simulink model "PubIfDecisionLSM_MDL"  (R2020b)
settings: configuration reference "DspaceConfig" (kept outside this file)
PostLoadFcn:
  | if any(exist('dsrtsu_mdlpostloadfcn', 'file') ~= 0), dsrtsu_mdlpostloadfcn('Execute', bdroot); end
InitFcn:
  | , if any(exist('rtifpga_mdlclblib', 'file') ~= 0), rtifpga_mdlclblib('Init', bdroot); end,
  | , if any(exist('dsmpb_private', 'file') ~= 0), dsmpb_private('dsmpb_mdlclblib', 'Init', bdroot); end,
values from neighbouring files (symbols this model uses):
  P_LSM_ALC_Enable = 0.0    [LSM_Parameter.sldd]
  P_LSM_AwayEdge_offset = 0.1    [LSM_Parameter.sldd]
  P_LSM_CentValidErr = 1.0    [LSM_Parameter.sldd]
  P_LSM_DOP_C0_EN_Limit = 0.8    [LSM_Parameter.sldd]
  P_LSM_DOP_C0_out_Limit = 2.0    [LSM_Parameter.sldd]
  P_LSM_DOP_C1_EN_Limit : value not decoded    [LSM_Parameter.sldd]
  P_LSM_DOP_C1_out_Limit : value not decoded    [LSM_Parameter.sldd]
  P_LSM_DOP_C1AndC2_Lim_X : value not decoded    [LSM_Parameter.sldd]
  P_LSM_DOP_C2_EN_Limit : value not decoded    [LSM_Parameter.sldd]
  P_LSM_DOP_C2_out_Limit : value not decoded    [LSM_Parameter.sldd]
  P_LSM_DOP_In_Pre2Dop_Dis = 1.0    [LSM_Parameter.sldd]
  P_LSM_DOP_Out_Pre2Dop_Dis = 2.0    [LSM_Parameter.sldd]
  P_LSM_DOP_PreDis_X : value not decoded    [LSM_Parameter.sldd]
  P_LSM_DOP_PreDis_Y : value not decoded    [LSM_Parameter.sldd]
  P_LSM_DOPEnableSW = 1.0    [LSM_Parameter.sldd]
  P_LSM_DOPValid_CheckTime = 0.06    [LSM_Parameter.sldd]
  P_LSM_DoubleLine_Curr2Cent_Dislimit = 0.5    [LSM_Parameter.sldd]
  P_LSM_DoubleLine_Dop2Cent_Dislimit = 0.5    [LSM_Parameter.sldd]
  P_LSM_DoubleLine_DOPOut_C1 : value not decoded    [LSM_Parameter.sldd]
  P_LSM_DoubleLine_Pre2Cent_Dislimit = 1.0    [LSM_Parameter.sldd]
  P_LSM_Error_Limit = 0.5    [LSM_Parameter.sldd]
  P_LSM_IFV2CenterAxis = 0.0    [LSM_Parameter.sldd]
  P_LSM_IFV2RearAxis = 0.0    [LSM_Parameter.sldd]
  P_LSM_Line2Edge_limit = 0.5    [LSM_Parameter.sldd]
  P_LSM_Line_Error = 0.1    [LSM_Parameter.sldd]
  P_LSM_LineSTD_Limit = 0.15    [LSM_Parameter.sldd]
  P_LSM_NOH_Switch = 0.0    [LSM_Parameter.sldd]
  P_LSM_OTL_C0_Factor = 1.0    [LSM_Parameter.sldd]
  P_LSM_OTL_C1_Factor = 0.5    [LSM_Parameter.sldd]
  P_LSM_OTL_C2_Factor = 0.5    [LSM_Parameter.sldd]
  P_LSM_Pre2OnlyLineDis = 5.0    [LSM_Parameter.sldd]
  P_LSM_Pre_t = 0.0    [LSM_Parameter.sldd]
  P_LSM_SingleLine_Cent2Edge_Dislimit = 100.0    [LSM_Parameter.sldd]
  P_LSM_SingleLine_Curr2Cent_Dislimit = 0.2    [LSM_Parameter.sldd]
  P_LSM_SingleLine_Dop2Cent_Dislimit = 0.2    [LSM_Parameter.sldd]
  P_LSM_SingleLine_DOPOut_C1 : value not decoded    [LSM_Parameter.sldd]
  P_LSM_SingleLine_Pre2Cent_Dislimit = 0.5    [LSM_Parameter.sldd]
  P_LSM_TJALimitSpd = 60.0    [LSM_Parameter.sldd]
undefined symbols (not defined in the file or in its folder): P_lCS_IFV2CenterAxis, P_LCS_IFV2RearAxis, P_LSM_EntryEdge_offset, P_LSM_EntryLnChngEnSwitch, P_LSM_EntryVanishDis, P_LSM_LinetLostTime, P_LSM_LineWijCal_C12, P_LSM_LineWijCal_C13, P_LSM_MapValid_ErrorSwitch, P_LSM_PosLineLcFac, P_LSM_SpdLim_Stub_Spd, P_LSM_SpdLim_StubLength, P_LSM_SpdTurnAlarm
libraries: simulink x324, TrueDurationTime x11
(part 15 of 25)

== matlab function PubIfDecisionLSM_MDL/Subsystem1/TargetLineCalc_20ms/TargetLineCalc/MATLAB Function4 ==
  data: LH1Wij input; LH2Wij input; LH1_Valid input; LH2_Valid input; CentLineValid output; VisLineConf input; VisLineA3 input; VisLineA2 input; VisLineA1 input; VisLineA0 input; VisLineR input; RoadWidth input; CentLineC3 output; CentLineC2 output; CentLineC1 output; CentLineC0 output; CentLineRange output; CentLineReliable output; LeftLineValid output; LeftLineC3 output; LeftLineC2 output; LeftLineC1 output; LeftLineC0 output; LeftLineRange output; LeftLineReliable output; LeftLaneAvail output; RightLineValid output; RightLineC3 output; RightLineC2 output; RightLineC1 output; RightLineC0 output; RightLineRange output; RightLineReliable output; RightLaneAvail output; Line_State output; preDis input
function [CentLineValid,CentLineC3,CentLineC2,CentLineC1,CentLineC0,CentLineRange,CentLineReliable,...
    LeftLineValid,LeftLineC3,LeftLineC2,LeftLineC1,LeftLineC0,LeftLineRange,LeftLineReliable,LeftLaneAvail,...
    RightLineValid,RightLineC3,RightLineC2,RightLineC1,RightLineC0,RightLineRange,RightLineReliable,RightLaneAvail,...
    Line_State] = ...
    VisFilter(LH1Wij,LH2Wij,LH1_Valid,LH2_Valid,...
    VisLineConf,VisLineA3,VisLineA2,VisLineA1,VisLineA0,VisLineR,RoadWidth,preDis)

CentLineValid = false;
CentLineC0 = single(0);
CentLineC1 = single(0);
CentLineC2 = single(0);
CentLineC3 = single(0);
CentLineRange = single(0);
CentLineReliable = single(0);
Line_State = uint8(0);

if (LH1_Valid) && (LH2_Valid)
    Range_Error = VisLineR(2) - VisLineR(3);
    LH1_Offset = single(0.5);
    LH2_Offset = single(0.5);
    if Range_Error>10 || Range_Error<-10
        LH1_Offset = 0.5+min(0.5,Range_Error*0.01);
        LH2_Offset = 1-LH1_Offset;
    end
    CentLineValid = true;
    CentLineC0 = 0.5*(VisLineA0(2) + VisLineA0(3));
    CentLineC1 = LH1_Offset*VisLineA1(2) + LH2_Offset*VisLineA1(3);
    CentLineC2 = LH1_Offset*VisLineA2(2) + LH2_Offset*VisLineA2(3);
    CentLineC3 = LH1_Offset*VisLineA3(2) + LH2_Offset*VisLineA3(3);
    CentLineRange = max(VisLineR(2),VisLineR(3));
    CentLineReliable = 0.5*(LH1Wij+LH2Wij);
    Line_State = uint8(3);
elseif LH1_Valid
    CentLineValid = true;
    CentLineC0 = VisLineA0(2)-0.5*RoadWidth*sqrt(1+VisLineA1(2)*VisLineA1(2));
    CentLineC1 = VisLineA1(2);
    CentLineC2 = VisLineA2(2);
    CentLineC3 = VisLineA3(2);
    CentLineRange = VisLineR(2);
    CentLineReliable = LH1Wij;
    Line_State = uint8(1);
elseif LH2_Valid
    CentLineValid = true;
    CentLineC0 = VisLineA0(3)+0.5*RoadWidth*sqrt(1+VisLineA1(3)*VisLineA1(3));
    CentLineC1 = VisLineA1(3);
    CentLineC2 = VisLineA2(3);
    CentLineC3 = VisLineA3(3);
    CentLineRange = VisLineR(3);
    CentLineReliable = LH2Wij;
    Line_State = uint8(2);
end

if LH1Wij>=0.3
    LeftLineValid = true;
    LeftLineC0 = VisLineA0(2) + 0.5*RoadWidth*sqrt(1+VisLineA1(2)*VisLineA1(2));
    LeftLineC1 = VisLineA1(2);
    LeftLineC2 = VisLineA2(2);
    LeftLineC3 = VisLineA3(2);
    LeftLineRange = VisLineR(2);
    LeftLineReliable = LH1Wij;
    t1 = VisLineA0(1)+VisLineA1(1)*preDis+VisLineA2(1)*preDis^2+VisLineA3(1)*preDis^3;
    t2 = VisLineA0(2)+VisLineA1(2)*preDis+VisLineA2(2)*preDis^2+VisLineA3(2)*preDis^3; 
    if (VisLineConf(1)>0)&&...
            ((VisLineA0(1)-VisLineA0(2))>3)&&...
            ((VisLineA0(1)-VisLineA0(2))<5.5)&&...
            ((t1 - t2)>3)
        LeftLaneAvail = true;
    else
        LeftLaneAvail = false;
    end
else
    LeftLineValid = false;
    LeftLineC0 = single(0);
    LeftLineC1 = single(0);
    LeftLineC2 = single(0);
    LeftLineC3 = single(0);
    LeftLineRange = single(0);
    LeftLineReliable = single(0);
    LeftLaneAvail = false;
end

if LH2Wij>=0.3
    RightLineValid = true;
    RightLineC0 = VisLineA0(3) - 0.5*RoadWidth*sqrt(1+VisLineA1(3)*VisLineA1(3));
    RightLineC1 = VisLineA1(3);
    RightLineC2 = VisLineA2(3);
    RightLineC3 = VisLineA3(3);
    RightLineRange = VisLineR(3);
    RightLineReliable = LH2Wij;
    
    t3 = VisLineA0(3)+VisLineA1(3)*preDis+VisLineA2(3)*preDis^2+VisLineA3(3)*preDis^3;
    t4 = VisLineA0(4)+VisLineA1(4)*preDis+VisLineA2(4)*preDis^2+VisLineA3(4)*preDis^3;

    if (VisLineConf(4)>0)&&...
            ((VisLineA0(3)-VisLineA0(4))>3)&&...
            ((VisLineA0(3)-VisLineA0(4))<5.5)&&...
            ((t3 - t4)>3)

        RightLaneAvail = true;
    else
        RightLaneAvail = false;
    end
else
    RightLineValid = false;
    RightLineC0 = single(0);
    RightLineC1 = single(0);
    RightLineC2 = single(0);
    RightLineC3 = single(0);
    RightLineRange = single(0);
    RightLineReliable = single(0);
    RightLaneAvail = false;
end

== matlab function PubIfDecisionLSM_MDL/Subsystem1/TargetLineCalc_20ms/TargetLineCalc/NOA ==
  data: LeftEn input boolean size=1; RightEn input boolean size=1; RFM_LineL1_Valid input uint8 size=1; RFM_LineL1_A0 input single size=1; RFM_LineL1_A1 input single size=1; RFM_LineL1_A2 input single size=1; RFM_LineL1_A3 input single size=1; RFM_LineL1_Range input single size=1; RFM_LineL2_Valid input uint8 size=1; RFM_LineL2_A0 input single size=1; RFM_LineL2_A1 input single size=1; RFM_LineL2_A2 input single size=1; RFM_LineL2_A3 input single size=1; RFM_LineL2_Range input single size=1; RFM_LineR1_Valid input uint8 size=1; RFM_LineR1_A0 input single size=1; RFM_LineR1_A1 input single size=1; RFM_LineR1_A2 input single size=1; RFM_LineR1_A3 input single size=1; RFM_LineR1_Range input single size=1; RFM_LineR2_Valid input uint8 size=1; RFM_LineR2_A0 input single size=1; RFM_LineR2_A1 input single size=1; RFM_LineR2_A2 input single size=1; RFM_LineR2_A3 input single size=1; RFM_LineR2_Range input single size=1; Exit_Valid input uint8 size=1; Exit_A0 input single size=1; Exit_A1 input single size=1; Exit_A2 input single size=1; Exit_A3 input single size=1; Exit_Range input single size=1; Exit_Start input; RFM_LineCL_Valid input uint8 size=1; RFM_LineCL_A0 input single size=1; RFM_LineCL_A1 input single size=1; RFM_LineCL_A2 input single size=1; RFM_LineCL_A3 input single size=1; RFM_LineCL_Range input single size=1; HWASts input uint8 size=1; HWAStsK1 input uint8 size=1; PilotSts input uint8 size=1; LaneChange input uint8 size=1; PilotRoadSts input uint8 size=1; DistanceLim input single size=1; HWALineValid output boolean size=1; MoveIDK1 input int8 size=1; HWALineC3 output single size=1; HWALineC2 output single size=1; HWALineC1 output single size=1; HWALineC0 output single size=1; HWARange output single size=1; HWALeLineValid output boolean size=1; HWALeLineC3 output single size=1; HWALeLineC2 output single size=1; HWALeLineC1 output single size=1; HWALeLineC0 output single size=1; HWALeRange output single size=1; HWARiLineValid output boolean size=1; HWARiLineC3 output single size=1; HWARiLineC2 output single size=1; HWARiLineC1 output single size=1; HWARiLineC0 output single size=1; HWARiRange output single size=1; MoveID output int8 size=1; LockIDK1 input int8 size=1; LockID output int8 size=1; Lock_counterK1 input uint8; Lock_counter output uint8
function [HWALineValid,HWALineC3,HWALineC2,HWALineC1,HWALineC0,HWARange,...
    HWALeLineValid,HWALeLineC3,HWALeLineC2,HWALeLineC1,HWALeLineC0,HWALeRange,...
    HWARiLineValid,HWARiLineC3,HWARiLineC2,HWARiLineC1,HWARiLineC0,HWARiRange,...
    MoveID,LockID,Lock_counter] = fcn(LeftEn,RightEn,RFM_LineL1_Valid,RFM_LineL1_A0,RFM_LineL1_A1,RFM_LineL1_A2,RFM_LineL1_A3,RFM_LineL1_Range,...
    RFM_LineL2_Valid,RFM_LineL2_A0,RFM_LineL2_A1,RFM_LineL2_A2,RFM_LineL2_A3,RFM_LineL2_Range,...
    RFM_LineR1_Valid,RFM_LineR1_A0,RFM_LineR1_A1,RFM_LineR1_A2,RFM_LineR1_A3,RFM_LineR1_Range,...
    RFM_LineR2_Valid,RFM_LineR2_A0,RFM_LineR2_A1,RFM_LineR2_A2,RFM_LineR2_A3,RFM_LineR2_Range,...
    Exit_Valid,Exit_A0,Exit_A1,Exit_A2,Exit_A3,Exit_Range,Exit_Start,...
    RFM_LineCL_Valid,RFM_LineCL_A0,RFM_LineCL_A1,RFM_LineCL_A2,RFM_LineCL_A3,RFM_LineCL_Range,HWASts,HWAStsK1,...
    PilotSts,LaneChange,PilotRoadSts,DistanceLim,MoveIDK1,LockIDK1,Lock_counterK1)
HWALineValid = false;
HWALineC3 = single(0);
HWALineC2 = single(0);
HWALineC1 = single(0);
HWALineC0 = single(0);
HWARange = single(0);

HWALeLineValid = false;
HWALeLineC3 = single(0);
HWALeLineC2 = single(0);
HWALeLineC1 = single(0);
HWALeLineC0 = single(0);
HWALeRange = single(0);

HWARiLineValid = false;
HWARiLineC3 = single(0);
HWARiLineC2 = single(0);
HWARiLineC1 = single(0);
HWARiLineC0 = single(0);
HWARiRange = single(0);

MoveID = MoveIDK1;
LockID = LockIDK1;
Lock_counter = max(Lock_counterK1-uint8(1),uint8(0));
if Lock_counter==0
    LockID = int8(0);
end

if (HWASts==1)||(HWASts==7)||(HWASts==0)||HWASts==2
    MoveID = int8(0);
end
Error=false;

%% NOH
if PilotSts~=0
    if HWASts==1||HWASts==2
        if RFM_LineCL_Valid>0
            HWALineValid = true;
            HWALineC3 = RFM_LineCL_A3;
            HWALineC2 = RFM_LineCL_A2;
            HWALineC1 = RFM_LineCL_A1;
            HWALineC0 = RFM_LineCL_A0;
            HWARange = RFM_LineCL_Range;
        end
        if RFM_LineL1_Valid>0&&RFM_LineL2_Valid>0&&...
                (RFM_LineL1_Range>DistanceLim||RFM_LineL2_Range>DistanceLim)&&LeftEn
            HWALeLineValid = true;
            HWALeLineC3 = 0.5*(RFM_LineL1_A3+RFM_LineL2_A3);
            HWALeLineC2 = 0.5*(RFM_LineL1_A2+RFM_LineL2_A2);
            HWALeLineC1 = 0.5*(RFM_LineL1_A1+RFM_LineL2_A1);
            HWALeLineC0 = 0.5*(RFM_LineL1_A0+RFM_LineL2_A0);
            HWALeRange = 0.5*(RFM_LineL1_Range+RFM_LineL2_Range);
        end
        if RFM_LineR1_Valid>0&&RFM_LineR2_Valid>0&&...
                (RFM_LineR1_Range>DistanceLim||RFM_LineR2_Range>DistanceLim)&&RightEn
            HWARiLineValid = true;
            HWARiLineC3 = 0.5*(RFM_LineR1_A3+RFM_LineR2_A3);
            HWARiLineC2 = 0.5*(RFM_LineR1_A2+RFM_LineR2_A2);
            HWARiLineC1 = 0.5*(RFM_LineR1_A1+RFM_LineR2_A1);
            HWARiLineC0 = 0.5*(RFM_LineR1_A0+RFM_LineR2_A0);
            HWARiRange = 0.5*(RFM_LineR1_Range+RFM_LineR2_Range);
        end
    end
    if PilotRoadSts==8&&Exit_Valid           %汇出（未行驶到汇出线）
        if Exit_Start>30
            HWALineValid = true;
            HWALineC3 = RFM_LineCL_A3;
            HWALineC2 = RFM_LineCL_A2;
            HWALineC1 = RFM_LineCL_A1;
            HWALineC0 = RFM_LineCL_A0;
            HWARange = RFM_LineCL_Range;
        elseif Exit_Start>16
            temp_x = [0.5*Exit_Start,Exit_Start,Exit_Start+single(10),Exit_Start+single(30)];
            y1 = RFM_LineCL_A0+RFM_LineCL_A1*temp_x(1)+RFM_LineCL_A2*temp_x(1)^2+RFM_LineCL_A3*temp_x(1)^3;
            y3 = Exit_A0+Exit_A1*temp_x(3)+Exit_A2*temp_x(3)^2+Exit_A3*temp_x(3)^3;
            if y3>0
                y2 = min(1,0.4*y3);
            else
                y2 = max(-1,0.4*y3);
            end
            y4 = Exit_A0+Exit_A1*temp_x(4)+Exit_A2*temp_x(4)^2+Exit_A3*temp_x(4)^3;
            temp_y = [y1,y2,y3,y4];
            [HWALineC3,HWALineC2,HWALineC1,HWALineC0] = pl(temp_x,temp_y);
            HWALineValid = true;
            HWARange = Exit_Start+single(40);
        else
            HWALineValid = true;
            HWALineC3 = Exit_A3;
            HWALineC2 = Exit_A2;
            HWALineC1 = Exit_A1;
            HWALineC0 = Exit_A0;
            HWARange = Exit_Range;
        end
    elseif PilotRoadSts==19&&Exit_Valid         % 汇出（行驶到汇出线）
        HWALineValid = true;
        HWALineC3 = Exit_A3;
        HWALineC2 = Exit_A2;
        HWALineC1 = Exit_A1;
        HWALineC0 = Exit_A0;
        HWARange = Exit_Range;
    elseif HWASts==3 || HWASts==11 || HWASts==12       %巡航
        MoveID = int8(0);
        if HWAStsK1==5 || HWAStsK1==6
            Lock_counter = uint8(250);
            LockID = int8(0);
        end
        if Lock_counter>0
            if LaneChange==1
                LockID = LockID + int8(1);
            end
            if LaneChange==2
                LockID = LockID - int8(1);
            end
        else
            LockID = int8(0);
        end
        if LockID==1
            if RFM_LineR1_Valid>0&&RFM_LineR2_Valid>0&&...
                    (RFM_LineR1_Range>DistanceLim||RFM_LineR2_Range>DistanceLim)
                HWALineValid = true;
                HWALineC3 = 0.5*(RFM_LineR1_A3+RFM_LineR2_A3);
                HWALineC2 = 0.5*(RFM_LineR1_A2+RFM_LineR2_A2);
                HWALineC1 = 0.5*(RFM_LineR1_A1+RFM_LineR2_A1);
                HWALineC0 = 0.5*(RFM_LineR1_A0+RFM_LineR2_A0);
                HWARange = 0.5*(RFM_LineR1_Range+RFM_LineR2_Range);
            elseif RFM_LineR1_Valid>0&&...
                    RFM_LineR1_Range>DistanceLim
                HWALineValid = true;
                HWALineC3 = RFM_LineR1_A3;
                HWALineC2 = RFM_LineR1_A2;
                HWALineC1 = RFM_LineR1_A1;
                HWALineC0 = RFM_LineR1_A0 - 1.875*sqrt(single(1) + RFM_LineR1_A1*RFM_LineR1_A1);
                HWARange = RFM_LineR1_Range;
            elseif RFM_LineR2_Valid>0&&...
                    RFM_LineR2_Range>DistanceLim
                HWALineValid = true;
                HWALineC3 = RFM_LineR2_A3;
                HWALineC2 = RFM_LineR2_A2;
                HWALineC1 = RFM_LineR2_A1;
                HWALineC0 = RFM_LineR2_A0 + 1.875*sqrt(single(1) + RFM_LineR2_A1*RFM_LineR2_A1);
                HWARange = RFM_LineR2_Range;
            end
        elseif LockID==-1
            if RFM_LineL1_Valid>0&&RFM_LineL2_Valid>0&&...
                    (RFM_LineL1_Range>DistanceLim||RFM_LineL2_Range>DistanceLim)
                HWALineValid = true;
                HWALineC3 = 0.5*(RFM_LineL1_A3+RFM_LineL2_A3);
                HWALineC2 = 0.5*(RFM_LineL1_A2+RFM_LineL2_A2);
                HWALineC1 = 0.5*(RFM_LineL1_A1+RFM_LineL2_A1);
                HWALineC0 = 0.5*(RFM_LineL1_A0+RFM_LineL2_A0);
                HWARange = 0.5*(RFM_LineL1_Range+RFM_LineL2_Range);
            elseif RFM_LineL1_Valid>0&&...
                    RFM_LineL1_Range>DistanceLim
                HWALineValid = true;
                HWALineC3 = RFM_LineL1_A3;
                HWALineC2 = RFM_LineL1_A2;
                HWALineC1 = RFM_LineL1_A1;
                HWALineC0 = RFM_LineL1_A0 - 1.875*sqrt(single(1) + RFM_LineL1_A1*RFM_LineL1_A1);
                HWARange = RFM_LineL1_Range;
            elseif RFM_LineL2_Valid>0&&...
                    RFM_LineL2_Range>DistanceLim
                HWALineValid = true;
                HWALineC3 = RFM_LineL2_A3;
                HWALineC2 = RFM_LineL2_A2;
                HWALineC1 = RFM_LineL2_A1;
                HWALineC0 = RFM_LineL2_A0 + 1.875*sqrt(single(1) + RFM_LineL2_A1*RFM_LineL2_A1);
                HWARange = RFM_LineL2_Range;
            end
        elseif LockID==0
            HWALineValid = true;
            HWALineC3 = RFM_LineCL_A3;
            HWALineC2 = RFM_LineCL_A2;
            HWALineC1 = RFM_LineCL_A1;
            HWALineC0 = RFM_LineCL_A0;
            HWARange = RFM_LineCL_Range;
        end
    elseif HWASts == 5                     %左换道
        if HWAStsK1~=5
            MoveID = MoveID - int8(1);
        end
        if LaneChange==1
            MoveID = MoveID + int8(1);
        end
        if LaneChange==2
            MoveID = MoveID - int8(1);
        end
        if (MoveID>=1)||(MoveID<=-2)
            Error = true;
        end
        if Error==false
            if MoveID==-1
                if RFM_LineL1_Valid>0&&RFM_LineL2_Valid>0&&...
                        (RFM_LineL1_Range>DistanceLim||RFM_LineL2_Range>DistanceLim)
                    HWALineValid = true;
                    HWALineC3 = 0.5*(RFM_LineL1_A3+RFM_LineL2_A3);
                    HWALineC2 = 0.5*(RFM_LineL1_A2+RFM_LineL2_A2);
                    HWALineC1 = 0.5*(RFM_LineL1_A1+RFM_LineL2_A1);
                    HWALineC0 = 0.5*(RFM_LineL1_A0+RFM_LineL2_A0);
                    HWARange = 0.5*(RFM_LineL1_Range+RFM_LineL2_Range);
                    
                    HWALeLineValid = true;
                    HWALeLineC3 = 0.5*(RFM_LineL1_A3+RFM_LineL2_A3);
                    HWALeLineC2 = 0.5*(RFM_LineL1_A2+RFM_LineL2_A2);
                    HWALeLineC1 = 0.5*(RFM_LineL1_A1+RFM_LineL2_A1);
                    HWALeLineC0 = 0.5*(RFM_LineL1_A0+RFM_LineL2_A0);
                    HWALeRange = 0.5*(RFM_LineL1_Range+RFM_LineL2_Range);
                elseif RFM_LineL1_Valid>0&&...
                        RFM_LineL1_Range>DistanceLim
                    HWALineValid = true;
                    HWALineC3 = RFM_LineL1_A3;
                    HWALineC2 = RFM_LineL1_A2;
                    HWALineC1 = RFM_LineL1_A1;
                    HWALineC0 = RFM_LineL1_A0 - 1.875*sqrt(single(1) + RFM_LineL1_A1*RFM_LineL1_A1);
                    HWARange = RFM_LineL1_Range;
                    
                    HWALeLineValid = true;
                    HWALeLineC3 = RFM_LineL1_A3;
                    HWALeLineC2 = RFM_LineL1_A2;
                    HWALeLineC1 = RFM_LineL1_A1;
                    HWALeLineC0 = RFM_LineL1_A0 - 1.875*sqrt(single(1) + RFM_LineL1_A1*RFM_LineL1_A1);
                    HWALeRange = RFM_LineL1_Range;
                elseif RFM_LineL2_Valid>0&&...
                        RFM_LineL2_Range>DistanceLim
                    HWALineValid = true;
                    HWALineC3 = RFM_LineL2_A3;
                    HWALineC2 = RFM_LineL2_A2;
                    HWALineC1 = RFM_LineL2_A1;
                    HWALineC0 = RFM_LineL2_A0 + 1.875*sqrt(single(1) + RFM_LineL2_A1*RFM_LineL2_A1);
                    HWARange = RFM_LineL2_Range;
                    HWALeLineValid = true;
                    HWALeLineC3 = RFM_LineL2_A3;
                    HWALeLineC2 = RFM_LineL2_A2;
                    HWALeLineC1 = RFM_LineL2_A1;
                    HWALeLineC0 = RFM_LineL2_A0 + 1.875*sqrt(single(1) + RFM_LineL2_A1*RFM_LineL2_A1);
                    HWALeRange = RFM_LineL2_Range;
                end
                HWARiLineValid = true;
                HWARiLineC3 = RFM_LineCL_A3;
                HWARiLineC2 = RFM_LineCL_A2;
                HWARiLineC1 = RFM_LineCL_A1;
                HWARiLineC0 = RFM_LineCL_A0;
                HWARiRange = RFM_LineCL_Range;
            elseif MoveID==0
                HWALineValid = true;
                HWALineC3 = RFM_LineCL_A3;
                HWALineC2 = RFM_LineCL_A2;
                HWALineC1 = RFM_LineCL_A1;
                HWALineC0 = RFM_LineCL_A0;
                HWARange = RFM_LineCL_Range;
            end
        end
    elseif HWASts==6                                     %右换道
        if HWAStsK1~=6
            MoveID = MoveID + int8(1);
        end
        if LaneChange==1
            MoveID = MoveID + int8(1);
        end
        if LaneChange==2
            MoveID = MoveID - int8(1);
        end
        if (MoveID>=2)||(MoveID<=-1)
            Error = true;
        end
        if Error==false
            if MoveID==1
                if RFM_LineR1_Valid>0&&RFM_LineR2_Valid>0&&...
                        (RFM_LineR1_Range>DistanceLim||RFM_LineR2_Range>DistanceLim)
                    HWALineValid = true;
                    HWALineC3 = 0.5*(RFM_LineR1_A3+RFM_LineR2_A3);
                    HWALineC2 = 0.5*(RFM_LineR1_A2+RFM_LineR2_A2);
                    HWALineC1 = 0.5*(RFM_LineR1_A1+RFM_LineR2_A1);
                    HWALineC0 = 0.5*(RFM_LineR1_A0+RFM_LineR2_A0);
                    HWARange = 0.5*(RFM_LineR1_Range+RFM_LineR2_Range);
                    
                    HWARiLineValid = true;
                    HWARiLineC3 = 0.5*(RFM_LineR1_A3+RFM_LineR2_A3);
                    HWARiLineC2 = 0.5*(RFM_LineR1_A2+RFM_LineR2_A2);
                    HWARiLineC1 = 0.5*(RFM_LineR1_A1+RFM_LineR2_A1);
                    HWARiLineC0 = 0.5*(RFM_LineR1_A0+RFM_LineR2_A0);
                    HWARiRange = 0.5*(RFM_LineR1_Range+RFM_LineR2_Range);
                elseif RFM_LineR1_Valid>0&&...
                        RFM_LineR1_Range>DistanceLim
                    HWALineValid = true;
                    HWALineC3 = RFM_LineR1_A3;
                    HWALineC2 = RFM_LineR1_A2;
                    HWALineC1 = RFM_LineR1_A1;
                    HWALineC0 = RFM_LineR1_A0 - 1.875*sqrt(single(1) + RFM_LineR1_A1*RFM_LineR1_A1);
                    HWARange = RFM_LineR1_Range;
                    
                    HWARiLineValid = true;
                    HWARiLineC3 = RFM_LineR1_A3;
                    HWARiLineC2 = RFM_LineR1_A2;
                    HWARiLineC1 = RFM_LineR1_A1;
                    HWARiLineC0 = RFM_LineR1_A0 - 1.875*sqrt(single(1) + RFM_LineR1_A1*RFM_LineR1_A1);
                    HWARiRange = RFM_LineR1_Range;
                elseif RFM_LineR2_Valid>0&&...
                        RFM_LineR2_Range>DistanceLim
                    HWALineValid = true;
                    HWALineC3 = RFM_LineR2_A3;
                    HWALineC2 = RFM_LineR2_A2;
                    HWALineC1 = RFM_LineR2_A1;
                    HWALineC0 = RFM_LineR2_A0 + 1.875*sqrt(single(1) + RFM_LineR2_A1*RFM_LineR2_A1);
                    HWARange = RFM_LineR2_Range;
                    HWARiLineValid = true;
                    HWARiLineC3 = RFM_LineR2_A3;
                    HWARiLineC2 = RFM_LineR2_A2;
                    HWARiLineC1 = RFM_LineR2_A1;
                    HWARiLineC0 = RFM_LineR2_A0 + 1.875*sqrt(single(1) + RFM_LineR2_A1*RFM_LineR2_A1);
                    HWARiRange = RFM_LineR2_Range;
                end
                HWALeLineValid = true;
                HWALeLineC3 = RFM_LineCL_A3;
                HWALeLineC2 = RFM_LineCL_A2;
                HWALeLineC1 = RFM_LineCL_A1;
                HWALeLineC0 = RFM_LineCL_A0;
                HWALeRange = RFM_LineCL_Range;
            elseif MoveID==0
                HWALineValid = true;
                HWALineC3 = RFM_LineCL_A3;
                HWALineC2 = RFM_LineCL_A2;
                HWALineC1 = RFM_LineCL_A1;
                HWALineC0 = RFM_LineCL_A0;
                HWARange = RFM_LineCL_Range;
            end
        end
    end
end

== matlab function PubIfDecisionLSM_MDL/Subsystem1/TargetLineCalc_20ms/TargetLineCalc/RoadWidthCalc1 ==
  data: YBranch_b input boolean size=1; VisLineConf input uint8 size=4; a1 input single size=4; a0 input single size=4; LineUpdate input boolean size=1; RoadWidth output single size=1; RoadWidthK1 input single size=1; tLostK1 input single size=1; tLost output single size=1
function [RoadWidth,tLost] = VisRoadWidth(YBranch_b,VisLineConf,a1,a0,LineUpdate,RoadWidthK1,tLostK1)

RoadWidth = RoadWidthK1;
tLost = tLostK1;
Update = false;
temp = single(0);

if LineUpdate
    if (VisLineConf(2)>0)&&(VisLineConf(3)>0)&&(YBranch_b==false)
        if abs(57.3*(atan(a1(2)) - atan(a1(3))))<3
            temp = (a0(2) - a0(3))/sqrt(a1(2)^2 + single(1));
            if (temp>2.5)&&(temp<4.2)
                Update = true;
            end
        end
    end
    if Update
        RoadWidth = 0.1*(temp - RoadWidthK1) + RoadWidthK1;
        tLost = single(0);
    else
        tLost = min(10,tLostK1 + single(0.05));
    end
end

== matlab function PubIfDecisionLSM_MDL/Subsystem1/TargetLineCalc_20ms/TargetLineCalc/MATLAB Function5 ==
  data: LH1Wij input; LH2Wij input; LH1_Valid output; LH2_Valid output; Wij_state output; kap input; preDis input; VisLineA3 input; VisLineA2 input; VisLineA1 input; VisLineA0 input
function [LH1_Valid,LH2_Valid,Wij_state] = fcn(LH1Wij,LH2Wij,...
    kap,preDis,VisLineA3,VisLineA2,VisLineA1,VisLineA0)

LH1_Valid = false;
LH2_Valid = false;
Wij_state = uint8(0);

dy_pre = 0.5*kap*preDis^2;
Curature2_pre = VisLineA1(2) + 2*VisLineA2(2)*preDis + 3*VisLineA3(2)*(preDis^2);
Curature3_pre = VisLineA1(3) + 2*VisLineA2(3)*preDis + 3*VisLineA3(3)*(preDis^2);
dy2 = (VisLineA0(2) + VisLineA1(2)*preDis + VisLineA2(2)*(preDis^2) + VisLineA3(2)*(preDis^3) - dy_pre)/sqrt(Curature2_pre^2+single(1));
dy3 = (VisLineA0(3) + VisLineA1(3)*preDis + VisLineA2(3)*(preDis^2) + VisLineA3(3)*(preDis^3) - dy_pre)/sqrt(Curature3_pre^2+single(1));
RoadWidth_Cur = VisLineA0(2)-VisLineA0(3);

if LH1Wij >= 0.3 && LH2Wij >= 0.3  %置信度都比较高
%     if LeftLightReq
%        LH1_Valid = true;
%        Wij_state = uint8(1);
%     elseif RightLightReq  %开启右转向
%         LH2_Valid = true;
%         Wij_state = uint8(2);
%     elseif StubValid>0 && StubStartDis<60 && (Direction==3 || Direction==1)  % 导航向左
%                 LH1_Valid = true;
%                 Wij_state = uint8(3);
%     elseif StubValid>0 && StubStartDis<60 && (Direction==4 || Direction==2)  % 导航向右
%                 LH2_Valid = true;
%                 Wij_state = uint8(4);
    
    if RoadWidth_Cur-(dy2-dy3)>0.5  || dy2-dy3-RoadWidth_Cur>0.5 ||...
            abs(VisLineA0(2) - VisLineA0(3))>4.2 ||...
            abs(VisLineA0(2) - VisLineA0(3))<2.6     %没方向，有分叉或过宽、过窄
        if LH1Wij >= LH2Wij
            LH1_Valid = true;
            Wij_state = uint8(3);
        else
            LH2_Valid = true;
            Wij_state = uint8(4);
        end
    else  %没方向，没分叉
        LH1_Valid = true;
        LH2_Valid = true;
        Wij_state = uint8(5);
    end
    
elseif LH1Wij >= 0.3 
    LH1_Valid = true;
    Wij_state = uint8(1);
elseif LH2Wij >= 0.3
    LH2_Valid = true;
    Wij_state = uint8(2);
end

== matlab function PubIfDecisionLSM_MDL/Subsystem1/TargetLineCalc_20ms/TargetLineCalc/MATLAB Function6 ==
  data: LeftOffset_b input boolean; RightOffset_b input boolean; LCKSts input; HWASts input; HWAStsK1 input; LaneChangeCancel_b output; LckLock_b output; Cnt1K1 input uint8; Cnt2K1 input uint8; Cnt1 output; Cnt2 output
function [LaneChangeCancel_b,LckLock_b,Cnt1,Cnt2] = ...
    fcn(LeftOffset_b,RightOffset_b,LCKSts,HWASts,HWAStsK1,Cnt1K1,Cnt2K1)

Cnt1 = max(Cnt1K1-uint8(1),uint8(0));
Cnt2 = max(Cnt2K1-uint8(1),uint8(0));

if HWASts==3 && (HWAStsK1==5||HWAStsK1==6)
    Cnt1 = uint8(250);
end

if Cnt1>0
    LaneChangeCancel_b = true;
else
    LaneChangeCancel_b = false;
end

if (LaneChangeCancel_b==false)&&...
        (HWASts~=5)&&(HWASts~=6)&&...
        (LCKSts==3)
   if LeftOffset_b || RightOffset_b
      Cnt2 = uint8(250);
   end
end

if LCKSts==1||LCKSts==0||LCKSts==2
    Cnt1 = uint8(0);
    Cnt2 = uint8(0);
end

if Cnt2>0
    LckLock_b = true;
else
    LckLock_b = false;
end

== stateflow chart PubIfDecisionLSM_MDL/Subsystem1/TargetLineCalc_20ms/TargetLineCalc/Subsystem3/Subsystem/Chart ==
  state init
    PilotRoadSts=PilotRoadSts_init;
  state init1
    PilotRoadSts=19;
  (default) -> init
  init -> init1 : [PilotRoadSts_init==19]
  init1 -> init : [bIsLineExist<2||rExitStub3==1||lExitStub3==1]
  data: PilotRoadSts_init input uint8 size=1; bIsLineExist input uint8 size=1; PilotRoadSts output uint8 size=1; lExitStub3 input boolean size=1; rExitStub3 input boolean size=1

== matlab function PubIfDecisionLSM_MDL/Subsystem1/TargetLineCalc_20ms/TargetLineCalc/LineSelect ==
  data: TJALineValid output boolean size=1; CentLaneValid input boolean size=1; CentLineA3 input single size=1; CentLineA2 input single size=1; CentLineA1 input single size=1; CentLineA0 input single size=1; CentRange input single size=1; OTLineValid input boolean size=1; aOTL input single size=1; bOTL input single size=1; cOTL input single size=1; dOTL input single size=1; dxMax input single size=1; TJA_Line_State input; TJALineA3 output single size=1; TJALineA2 output single size=1; TJALineA1 output single size=1; TJALineA0 output single size=1; TJALineRange output single size=1; LCKLineValid output boolean size=1; LCKLineA3 output single size=1; LCKLineA2 output single size=1; LCKLineA1 output single size=1; LCKLineA0 output single size=1; LCKLineRange output single size=1
function [TJALineValid,TJALineA3,TJALineA2,TJALineA1,TJALineA0,TJALineRange,...
    LCKLineValid,LCKLineA3,LCKLineA2,LCKLineA1,LCKLineA0,LCKLineRange] = ...
    LineSelect(CentLaneValid,CentLineA3,CentLineA2,CentLineA1,CentLineA0,CentRange,...
    OTLineValid,aOTL,bOTL,cOTL,dOTL,dxMax,TJA_Line_State)

TJALineValid = false;
TJALineA3 = single(0);
TJALineA2 = single(0);
TJALineA1 = single(0);
TJALineA0 = single(0);
TJALineRange = single(0);

if (CentLaneValid==true)&&(CentRange>12)
    LCKLineValid = true;
    LCKLineA3 = CentLineA3;
    LCKLineA2 = CentLineA2;
    LCKLineA1 = CentLineA1;
    LCKLineA0 = CentLineA0;
    LCKLineRange = CentRange;
else
    LCKLineValid = false;
    LCKLineA3 = single(0);
    LCKLineA2 = single(0);
    LCKLineA1 = single(0);
    LCKLineA0 = single(0);
    LCKLineRange = single(0);
end

% TJALimitSpd = 20;
% temp = (TJALimitSpd - 1.3)/1.03;
% temp = temp/3.6;


if TJA_Line_State == 1 || TJA_Line_State == 0
   
    TJALineValid = CentLaneValid;
    TJALineA3 = CentLineA3;
    TJALineA2 = CentLineA2;
    TJALineA1 = CentLineA1;
    TJALineA0 = CentLineA0;
    TJALineRange = CentRange;
elseif TJA_Line_State == 2
    TJALineValid = OTLineValid;
    TJALineA3 = aOTL;
    TJALineA2 = bOTL;
    TJALineA1 = cOTL;
    TJALineA0 = dOTL;
    TJALineRange = dxMax;
end
